simulink model "lab2sim"  (R2015b)
settings: Solver=ode4  StartTime=0.0  StopTime=0.002  FixedStep=0.0000002  RelTol=1e-3
values from neighbouring files (symbols this model uses):
  b = 50    [script1.m]
  k = 2e5    (= 200000)    [script1.m]
  Kf = 2*pi*r*N*B    (= 3.14159265359)    [script1.m]
  L = 0.05e-3    (= 5e-05)    [script1.m]
  m = 4e-3    (= 0.004)    [script1.m]
  R = 5    [script1.m]
settings Model: ExtModeTrigDuration=10000  Creator=husseinz  LastModifiedBy=husseinz
settings SolverCC: PositivePriorityOrder=on
settings RTWCC: SystemTargetFile=quarc_win64.tlc  TemplateMakefile=quarc_default_tmf  Description=QUARC Win64 Target
settings STFCustomTargetCC: TargetPreCompLibLocation=C:\ProgramData\QUARC\lib\2015b\win64\release  GeneratePreprocessorConditionals=Use local settings  CPPClassGenCompliant=off
settings GRTTargetCC: TargetPreCompLibLocation=C:\ProgramData\QUARC\lib\2015b\win64\release  ParMdlRefBuildCompliant=off  CompOptLevelCompliant=off  CombineOutputUpdateFcns=off  MatFileLogging=off  CPPClassGenCompliant=off  GRTInterface=on  UseToolchainInfoCompliant=off  ExtMode=on  ExtModeMexFile=quarc_comm

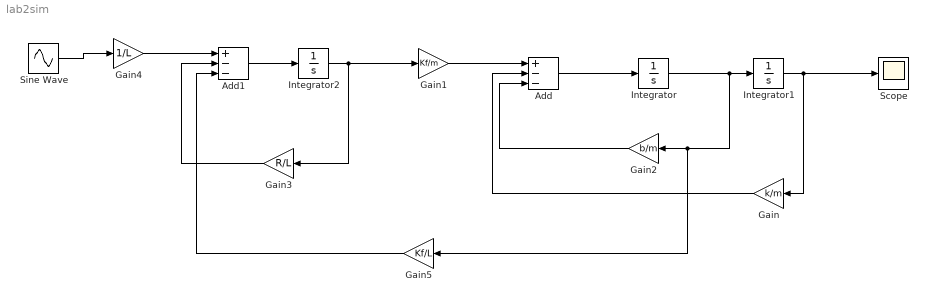
== system lab2sim ==
  Add : Sum  Inputs=+--
  Add1 : Sum  Inputs=+--
  Gain : Gain  Gain=k/m
  Gain1 : Gain  Gain=Kf/m
  Gain2 : Gain  Gain=b/m
  Gain3 : Gain  Gain=R/L
  Gain4 : Gain  Gain=1/L
  Gain5 : Gain  Gain=Kf/L
  Integrator : Integrator
  Integrator1 : Integrator
  Integrator2 : Integrator
  Scope : Scope
  Sine Wave : Sin  Frequency=20000  SampleTime=0
  wires:
  Add/1 -> Integrator/1
  Integrator/1 -> Gain5/1, Gain2/1, Integrator1/1
  Integrator1/1 -> Scope/1, Gain/1
  Gain1/1 -> Add/1
  Gain/1 -> Add/2
  Gain2/1 -> Add/3
  Add1/1 -> Integrator2/1
  Integrator2/1 -> Gain1/1, Gain3/1
  Gain3/1 -> Add1/2
  Gain4/1 -> Add1/1
  Sine Wave/1 -> Gain4/1
  Gain5/1 -> Add1/3
